simulink model "laplace_pid_closed_loop"  (R2026a)
settings: Solver=FixedStepDiscrete  StopTime=11.99  FixedStep=0.01

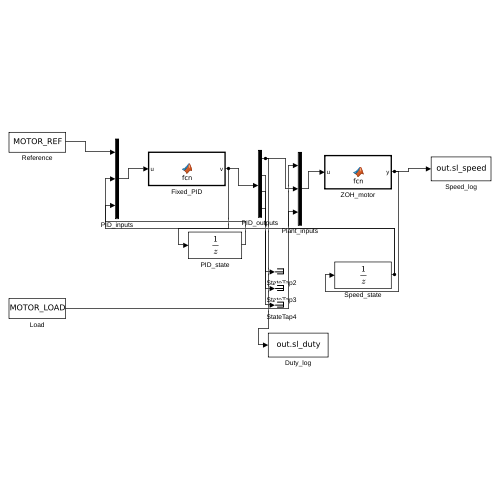
[thumbnail: Simulink's stored preview of the top-level diagram]
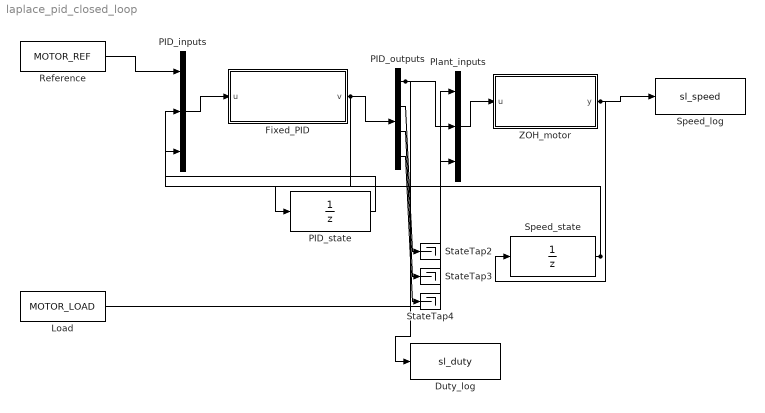
== system laplace_pid_closed_loop ==
  Duty_log : ToWorkspace  VariableName=sl_duty  SampleTime=-1
  Fixed_PID : MATLAB Function  TreatAsAtomicUnit=on
  Load : FromWorkspace  VariableName=MOTOR_LOAD  Interpolate=off  OutputAfterFinalValue=Holding final value
  PID_inputs : Mux  Inputs=3
  PID_outputs : Demux
  PID_state : UnitDelay  InitialCondition=[0;0;0;0]  SampleTime=0.01
  Plant_inputs : Mux  Inputs=3
  Reference : FromWorkspace  VariableName=MOTOR_REF  Interpolate=off  OutputAfterFinalValue=Holding final value
  Speed_log : ToWorkspace  VariableName=sl_speed  SampleTime=-1
  Speed_state : UnitDelay  SampleTime=0.01
  StateTap2 : Terminator
  StateTap3 : Terminator
  StateTap4 : Terminator
  ZOH_motor : MATLAB Function  TreatAsAtomicUnit=on
  wires:
  Reference/1 -> PID_inputs/1
  Speed_state/1 -> PID_inputs/2, Plant_inputs/1
  PID_state/1 -> PID_inputs/3
  PID_inputs/1 -> Fixed_PID/1(u)
  Fixed_PID/1(v) -> PID_state/1, PID_outputs/1
  PID_outputs/1 -> Plant_inputs/2, Duty_log/1
  Load/1 -> Plant_inputs/3
  Plant_inputs/1 -> ZOH_motor/1(u)
  ZOH_motor/1(y) -> Speed_state/1, Speed_log/1
  PID_outputs/2 -> StateTap2/1
  PID_outputs/3 -> StateTap3/1
  PID_outputs/4 -> StateTap4/1

== matlab function laplace_pid_closed_loop/Fixed_PID ==
  data: u input; v output
function v=fcn(u)
v=pid_sl(u);
end

== matlab function laplace_pid_closed_loop/ZOH_motor ==
  data: u input; y output
function y=fcn(u)
a=61258;
y=floor((a*u(1)+(65536-a)*max(u(2)-u(3),0))/65536);
end
